simulink model "MS_QD2_QBPlat_R2021a"  (R2021a)
settings: Solver=ode2  StartTime=0.0  StopTime=inf  FixedStep=0.001  RelTol=1e-3  EnableMultiTasking=on
undefined symbols (not defined in the file): Host, localhost, qc_get_step_size
libraries: quarc_library x71, simulink x10, simulink_extras x2
(part 1 of 2)
settings Model: SimulationMode=external  ExtModeTrigDuration=10000  Creator=Admin  LastModifiedBy=jpineros
settings SolverCC: AlgebraicLoopSolver=TrustRegion  PositivePriorityOrder=on
settings DataIOCC: ReturnWorkspaceOutputs=off
settings DebuggingCC: SFUnexpectedBacktrackingDiag=warning  SFNoUnconditionalDefaultTransitionDiag=warning  SFExecutionAtInitializationDiag=none  ArithmeticOperatorsInVariantConditions=warning
settings SFSimCC: SimUseLocalCustomCode=off  CustomCodeUndefinedFunction=UseInterfaceOnly
settings RTWCC: Description=QUARC Win64 Target Using Toolchain  SystemTargetFile=quarc_win64.tlc  TemplateMakefile=quarc_default_tmf  RTWUseLocalCustomCode=off  Toolchain=QUARC win64 | nmake (64-bit Windows)  BuildConfiguration=Faster Runs
settings CodeAppCC: StateflowObjectComments=on
settings STFCustomTargetCC: ConcurrentExecutionCompliant=on  SystemTargetFile=quarc_win64.tlc
settings GRTTargetCC: TargetLangStandard=C89/C90 (ANSI)  ParMdlRefBuildCompliant=off  CompOptLevelCompliant=off  CombineOutputUpdateFcns=off  MatFileLogging=off  CPPClassGenCompliant=off  GRTInterface=on  ExtMode=on  ExtModeMexFile=quarc_comm  ExtModeMexArgs='-w -d %d -uri %u -drone_ip 192.168.2.11 -qbot_ip 192.168.2.21','tcpip://localhost:17001'
settings ConfigComp: CovMetricSettings=dw  CovSaveCumulativeToWorkspaceVar=on  CovSaveSingleToWorkspaceVar=on  CovExternalEMLEnable=off  CovBoundaryAbsTol=1.0e-5

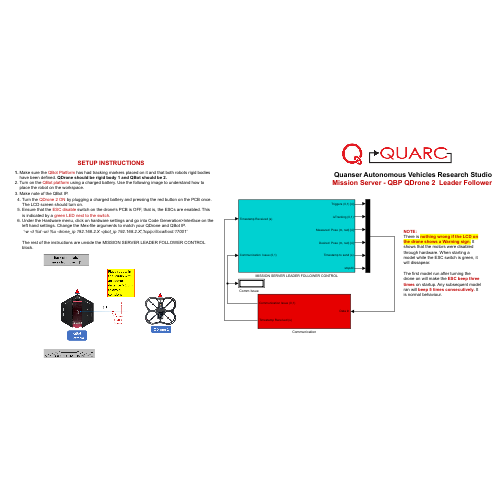
[thumbnail: Simulink's stored preview of the top-level diagram]
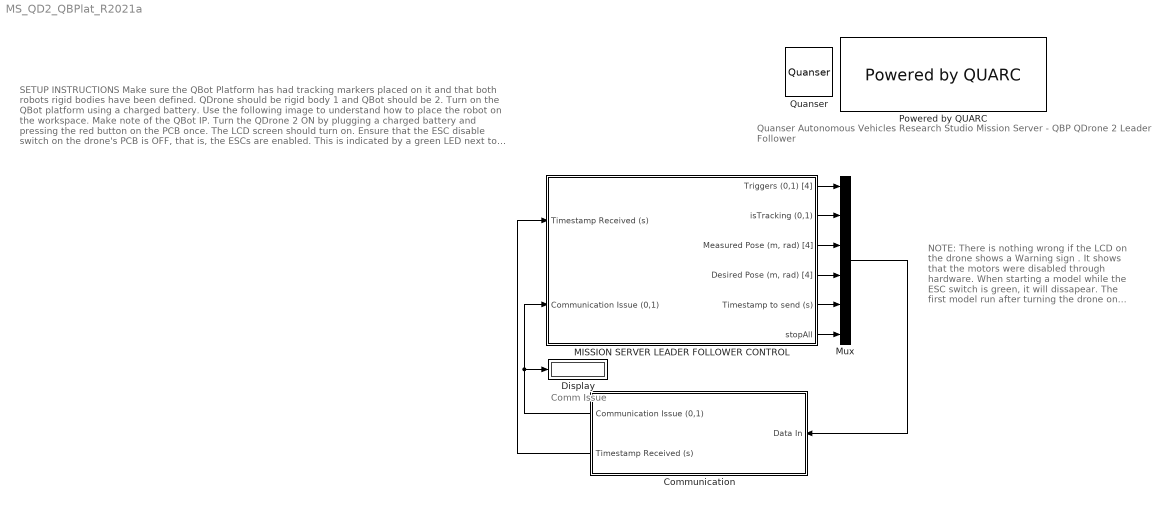
== system MS_QD2_QBPlat_R2021a ==
  note: Quanser Autonomous Vehicles Research Studio
      | Mission Server - QBP QDrone 2 Leader Follower
  note: Comm Issue
  note: NOTE:
      | There is nothing wrong if the LCD on the drone shows a Warning sign . It shows that the motors were disabled through hardware. When starting a model while the ESC switch is green, it will dissapear.
      |
      | The first model run after turning the drone on will make the ESC beep three times on startup. Any subsequent model ran will beep 5 times consecutively. It is normal behaviour.
  note: SETUP INSTRUCTIONS
      |
      | Make sure the QBot Platform has had tracking markers placed on it and that both robots rigid bodies have been defined. QDrone should be rigid body 1 and QBot should be 2.
      | Turn on the QBot platform using a charged battery. Use the following image to understand how to place the robot on the workspace.
      | Make note of the QBot IP.
      | Turn the QDrone 2 ON by plugging a charged battery and pressing the red button on the PCB once. The LCD screen should turn on.
      | Ensure that the ESC disable switch on the drone's PCB is OFF, that is, the ESCs are enabled. This is indicated by a green LED next to the switch .
      | Under the Hardware menu, click on hardware settings and go into Code Generation>Interface on the left hand settings. Change the Mex-file arguments to match your QDrone and QBot IP.
      | '-w -d %d -uri %u -drone_ip 192.168.2.X -qbot_ip 192.168.2.X','tcpip://localhost:17001'
      |
      | The rest of the instructions are unside the MISSION SERVER LEADER FOLLOWER CONTROL block.
  Communication : Subsystem
  Display : Display
  MISSION SERVER LEADER FOLLOWER CONTROL : Subsystem
  Mux : Mux  Inputs=6
  Powered by QUARC : quarc_library/Logos/Powered by QUARC
  Quanser : quarc_library/Logos/Quanser
  wires:
  Communication/2(Timestamp Received (s)) -> MISSION SERVER LEADER FOLLOWER CONTROL/1(Timestamp Received (s))
  MISSION SERVER LEADER FOLLOWER CONTROL/5(Timestamp to send (s)) -> Mux/5
  Mux/1 -> Communication/1(Data In)
  Communication/1(Communication Issue (0,1)) -> MISSION SERVER LEADER FOLLOWER CONTROL/2(Communication Issue (0,1)), Display/1
  MISSION SERVER LEADER FOLLOWER CONTROL/3("Measured Pose (m, rad) [4]") -> Mux/3
  MISSION SERVER LEADER FOLLOWER CONTROL/4("Desired Pose (m, rad) [4]") -> Mux/4
  MISSION SERVER LEADER FOLLOWER CONTROL/1(Triggers (0,1) [4]) -> Mux/1
  MISSION SERVER LEADER FOLLOWER CONTROL/2(isTracking (0,1)) -> Mux/2
  MISSION SERVER LEADER FOLLOWER CONTROL/6(stopAll) -> Mux/6

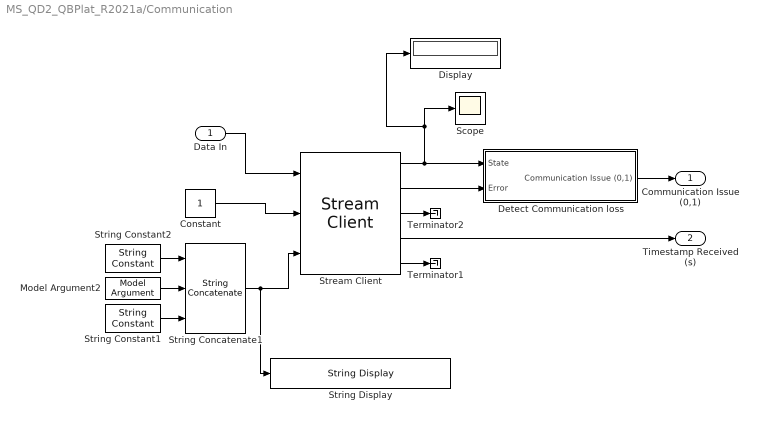
== system MS_QD2_QBPlat_R2021a/Communication ==
  Data In : Inport
  Constant : Constant
  Detect Communication loss : Subsystem
  Display : Display
  Model Argument2 : quarc_library/Sources/Signals/Model Argument  argument_name=drone_ip  has_value=on  data_type_mode=Specify via dialog  data_type=char  max_length=80  default_value=0  default_string=192.168.2.11  variable_size=off
      settings: AttributesFormatString=(-%<argument_name>)  SourceProductName=QUARC Targets
  Scope : Scope
  Stream Client : quarc_library/Communications/Basic/Stream Client  uri_source=External input port  uri=tcpip://192.168.2.11:18011  send_buffer_size=1460  receive_buffer_size=1460  byte_order=little endian (Intel - LSB first)  optimization=Minimum latency  send_options=Send most recent data  receive_options=Receive most recent data  default_value=zeros(1,1)  sample_time=qc_get_step_size  active=off  implementation=Use blocking I/O in a separate thread  send_fifo_size=1000  receive_fifo_size=1000  send_priority=0  receive_priority=0  send_dimensions=off  receive_dimensions=off  max_dimensions=-1  data_type=Inherited via back propagation  type_expr=BusObject
  String Concatenate1 : quarc_library/Strings/String Concatenate  num_inputs=3  max_length=0  output_size=Inherit from input
      settings: SourceProductName=QUARC Targets
  String Constant1 : quarc_library/Strings/String Constant  string_value=:18011?nagle='off'  evaluate_string=off  string_type=text  max_length=80  sample_time=inf  variable_size=off
      settings: AttributesFormatString="\":18011?nagle='off'\""  SourceProductName=QUARC Targets
  String Constant2 : quarc_library/Strings/String Constant  string_value=tcpip://  evaluate_string=off  string_type=text  max_length=80  sample_time=inf  variable_size=off
      settings: AttributesFormatString="\"tcpip://\""  SourceProductName=QUARC Targets
  String Display : quarc_library/Strings/String Display  alignment=center  display_mode=Single line  sample_time=-1  use_new=off
      settings: SourceProductName=QUARC Targets
  Terminator1 : Terminator
  Terminator2 : Terminator
  Communication Issue (0,1) : Outport  VectorParamsAs1DForOutWhenUnconnected=off
  Timestamp Received (s) : Outport  Port=2  VectorParamsAs1DForOutWhenUnconnected=off
  wires:
  Constant/1 -> Stream Client/2
  Data In/1 -> Stream Client/1
  Stream Client/3 -> Terminator2/1
  Stream Client/5 -> Terminator1/1
  Stream Client/4 -> Timestamp Received (s)/1
  Stream Client/1 -> Display/1, Scope/1, Detect Communication loss/1(State)
  Stream Client/2 -> Detect Communication loss/2(Error)
  Detect Communication loss/1(Communication Issue (0,1)) -> Communication Issue (0,1)/1
  Model Argument2/1 -> String Concatenate1/2
  String Constant2/1 -> String Concatenate1/1
  String Concatenate1/1 -> Stream Client/3, String Display/1
  String Constant1/1 -> String Concatenate1/3

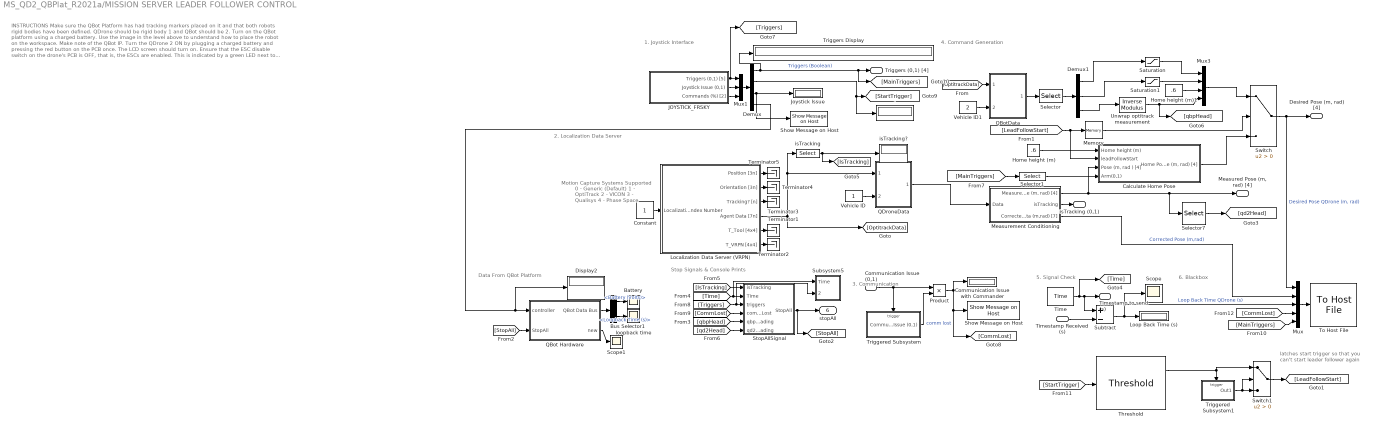
== system MS_QD2_QBPlat_R2021a/MISSION SERVER LEADER FOLLOWER CONTROL ==
  note: Data From QBot Platform
  note: Stop Signals & Console Prints
  note: latches start trigger so that you can't start leader follower again
  note: 5. Signal Check
  note: 6. Blackbox
  note: 3. Communication
  note: 2. Localization Data Server
  note: 1. Joystick Interface
  note: 4. Command Generation
  note: INSTRUCTIONS
      |
      | Make sure the QBot Platform has had tracking markers placed on it and that both robots rigid bodies have been defined. QDrone should be rigid body 1 and QBot should be 2.
      | Turn on the QBot platform using a charged battery. Use the image in the level above to understand how to place the robot on the workspace.
      | Make note of the QBot IP.
      | Turn the QDrone 2 ON by plugging a charged battery and pressing the red button on the PCB once. The LCD screen should turn on.
      | Ensure that the ESC disable switch on the drone's PCB is OFF, that is, the ESCs are enabled. This is indicated by a green LED next to the switch .
      | Under the Hrdware menu, click on hardware settings and go into Code Generation>Interface on the left hand settings. Change the Mex-file arguments to match your QDrone and QBot IP.
      | '-w -d %d -uri %u -drone_ip 192.168.2.X -qbot_ip 192.168.2.X','tcpip://localhost:17001'
      |
      | Open the Joystick subsystem and ensure that the Host Game Controller block's Controller Number parameter is set to FrSky Simulator THAT SUBSYSTEM ALSO WILL SHOW YOU HOW TO CONTROL THE SYSTEM USING THE DIFFERENT PARTS OF THE JOYSTICK
      | NOTE : In case of unexpected behaviour or emergencies, keep the Emergency Stop push button pressed on the joystick to cut all power to the motors (this will result in the drone falling).
      | Localization subsystem uses VRPN to communicate with third party motion capture systems. Change the motion capture system selector to the one currently used by your lab. Systems currently tested:
      | 0 - Generic (Default)
      | 1 - OptiTrack
      | 2 - VICON
      | 3 - Qualisys
      | 4 - Phase Space
      | Note: DO NOT change this number once the model has started.
      | Turn the Joystick ON and ensure all toggles are on the position away from you .
      | Under the HARDWARE menu, click on Monitor & Tune . Wait for the model to start running (takes ~1 to 5 seconds for the Motive API to initialize and send localization data).
      | In the MISSION CONTROL QDRONE POSITION CONTROL subsystem, ensure that the isTracking? display shows both values as 1 and that the Joystick Issue display shows 0 (joystick must be powered ON with USB dongle attached to the PC).
      | In your file explorer in the same folder as this file, right click on qbot_driver.rt-linux_qbot_platform and click on run on target.
      | Fill out the window that pops up as per the image underneath using the IP in the QBot's screen and click run. The LEDs of the QBot should changeto white.
      | Note: If you are used to running the qbot driver on startup for the QBot, stop the model and run this one instead. It has some modifications from the default QBot driver in other examples.
      | You should now be able to drive the QBot using the right joystick on the controller.
      |
      | In a new Matlab instance, open the QDrone.slx model and set the QDrone's IP in the Hardware Settings > Code Generation > Interface and click Monitor and drone. Wait for the Drone to beep.
      | Arm the drone by moving the Arm/Disarm toggle on the joystick to the 2 position. (Bringing it towards you). The props will start turning at a low speed.
      | Takeoff the drone by moving the Takeoff/Land toggle on the joystick to the 2 position (Bringing it towards you). The QDrone should takeoff and hover.
      | Switch the Leader Follower Start toggle (toggle on the right front of the joystick, use the image inside the joystick subsystem as a reference) towards you and the QDrone will start following above the QBot.
      | Drive the QBot with the joystick in the controller. The drone will fly only 1 meter on each direction of the origin, so if the qbot exits that area, the QDrone will stay behind but pointed towards the qbot.
      | Once done, switch the Leader follower Start toggle back to the starting position away from you and the QDrone will stay at its current position. Use the joystick to move the QBot away from under the QDrone.
      | When the QBot is safely away from the Drone, move the Takeoff/Land toggle on the joystick to the 0 position to land the drone. The QDrone should land.
      | Move the Arm/Disarm toggle on the joystick to the 0 position. (The QDrone.slx model disarms the drone and stops automatically upon landing).
      | Stop this model.
  note: Motion Capture Systems Supported
  note: 0 - Generic (Default)
      | 1 - OptiTrack
      | 2 - VICON
      | 3 - Qualisys
      | 4 - Phase Space
  Timestamp Received (s) : Inport
  Communication Issue (0,1) : Inport  Port=2
  . : Display
  Battery : Scope
  Bus Selector1 : BusSelector  OutputSignals=Battery (Volts),Loopback Time (s)
  Calculate Home Pose : Subsystem
  Communication Issue with Commander : Display
  Constant : Constant
  Demux : Demux  Outputs=[4 1 1 2]
  Demux1 : Demux  Outputs=3
  Display2 : Display
  Home height (m) : Constant  Value=.6
  Home height (m)1 : Constant  Value=.6
  JOYSTICK_FRSKY : Subsystem
      mask Display: image('frsky.jpg');
  Joystick Issue : Display
  "Localization Data Server (VRPN) " : Subsystem
  Loop Back Time (s) : Display
  Measurement Conditioning : Subsystem
  Memory : Memory
  Mux : Mux  Inputs=5
  Mux1 : Mux  Inputs=[5 1 2]
  Mux3 : Mux
  Product : Product
  QBot Hardware : Subsystem
  QBotData : Subsystem
  QDroneData : Subsystem
  Saturation : Saturate  UpperLimit=1  LowerLimit=-1
  Saturation1 : Saturate  UpperLimit=1  LowerLimit=-1
  Scope : Scope
  Scope1 : Scope
  Selector : Selector  InputPortWidth=7  IndexOptions=Index vector (dialog)  Indices=[1 2 6]  OutputSizes=1
  Selector1 : Selector  InputPortWidth=4  IndexOptions=Index vector (dialog)  Indices=[1]  OutputSizes=1
  Selector7 : Selector  InputPortWidth=4  IndexOptions=Index vector (dialog)  Indices=[4]  OutputSizes=1
  Show Message on Host : quarc_library/Sinks/Error Handling/Show Message on Host  message_type=Fixed error message  message_icon=Warning  message=Mission Server: Communication Issue with QDrone
      settings: AttributesFormatString="\"%<message>\""  SourceProductName=QUARC Targets
  "Show Message on Host " : quarc_library/Sinks/Error Handling/Show Message on Host  message_type=Fixed error message  message_icon=Warning  message=Mission Server: Joystick Disconnected
      settings: AttributesFormatString="\"%<message>\""  SourceProductName=QUARC Targets
  StopAllSignal : Subsystem
  Subsystem5 : Subsystem
  Subtract : Sum  Inputs=+-
  Switch : Switch  Criteria=u2 > Threshold
  Switch1 : Switch  Criteria=u2 > Threshold
  Terminator{1..5} (5 alike) : Terminator
  Threshold : quarc_library/Discontinuities/Threshold  operator=>  param_src=Specify via dialog  threshold=0  duration=0.1
      settings: SourceProductName=QUARC Targets
  Time : quarc_library/Sources/Time/Time  time_source=Wall clock  sample_time=qc_get_step_size
  To Host File : quarc_library/Sinks/To Host/To Host File  source=Specify via dialog (do not evaluate)  file_name=saved_data/%m/Mission_Server_%{date}_%{time}.mat  variable_name=mission_server_data  decimation=1  sample_time=-1  file_format=MAT-file v.5  options=No header or footer  append=off  final_file_name=saved_data/MS_QD2_QBPlat_R2021a_/Mission_Server_30-Sep-2026_09-51-03.mat  encoding=Default  bitrate=2000000
  Triggered Subsystem1 : Subsystem  TreatAsAtomicUnit=on
  Triggered Subsystem : Subsystem  TreatAsAtomicUnit=on
  Triggers Display : Display
  Unwrap optitrack measurement : quarc_library/Discontinuities/Inverse Modulus  modulus=2*pi  output_derivative=off  output_revolutions=off  max_x=Inf  min_x=-Inf
  Vehicle ID : Constant
  Vehicle ID1 : Constant  Value=2
  isTracking : Selector  InputPortWidth=14  IndexOptions=Index vector (dialog)  Indices=[7 14]  OutputSizes=1
  isTracking? : Display
  loopback time : Scope
  Triggers (0,1) [4] : Outport  VectorParamsAs1DForOutWhenUnconnected=off
  isTracking (0,1) : Outport  Port=2  VectorParamsAs1DForOutWhenUnconnected=off
  "Measured Pose (m, rad) [4]" : Outport  Port=3  VectorParamsAs1DForOutWhenUnconnected=off
  "Desired Pose (m, rad) [4]" : Outport  Port=4  VectorParamsAs1DForOutWhenUnconnected=off
  Timestamp to send (s) : Outport  Port=5  VectorParamsAs1DForOutWhenUnconnected=off
  stopAll : Outport  Port=6
  wires:
  Communication Issue (0,1)/1 -> Product/1, Triggered Subsystem/Trigger
  isTracking/1 -> isTracking?/1, [IsTracking]
  Demux/3 -> Joystick Issue/1, "Show Message on Host "/1
  Demux/1 -> Triggers (0,1) [4]/1, [MainTriggers], Triggers Display/1  "Triggers (Boolean)"
  Time/1 -> [Time], Subtract/1, Timestamp to send (s)/1
  Timestamp Received (s)/1 -> Subtract/2
  Subtract/1 -> Mux/3, Scope/1, Loop Back Time (s)/1  "Loop Back Time QDrone (s)"
  Switch/1 -> Mux/1, "Desired Pose (m, rad) [4]"/1  "Desired Pose QDrone (m, rad)"
  Measurement Conditioning/2(isTracking) -> isTracking (0,1)/1
  Vehicle ID/1 -> QDroneData/2(Vehicle ID)
  QDroneData/1(Vehicle Data) -> Measurement Conditioning/1(Data)
  Home height (m)/1 -> Calculate Home Pose/1(Home height (m))
  Triggered Subsystem/1(Communication Issue (0,1)) -> Product/2
  Product/1 -> Communication Issue with Commander/1, [CommLost], Show Message on Host/1  "comm lost"
  Mux/1 -> To Host File/1
  Selector1/1 -> Calculate Home Pose/4(Arm(0,1))
  Measurement Conditioning/1("Measured Pose (m, rad) [4]") -> Calculate Home Pose/3("Pose (m, rad ) [4]"), "Measured Pose (m, rad) [4]"/1, Selector7/1
  Measurement Conditioning/3(Corrected Pose Data (m,rad) [7]) -> Mux/2  "Corrected Pose (m,rad)"
  Mux1/1 -> Demux/1
  Calculate Home Pose/1("Home Pose (m, rad) [4]") -> Switch/3
  [LeadFollowStart] -> Calculate Home Pose/2(leadFollowStart), Memory/1
  JOYSTICK_FRSKY/2(Joystick Issue (0,1)) -> Mux1/2
  JOYSTICK_FRSKY/1(Triggers (0,1) [5]) -> [Triggers], Mux1/1
  JOYSTICK_FRSKY/3(Commands (%) [2]) -> Mux1/3
  Vehicle ID1/1 -> QBotData/2(Vehicle ID)
  QBotData/1(Vehicle Data) -> Selector/1
  Selector/1 -> Demux1/1
  Demux1/1 -> Saturation/1
  Demux1/2 -> Saturation1/1
  Demux1/3 -> Unwrap optitrack measurement/1
  Home height (m)1/1 -> Mux3/3
  Mux3/1 -> Switch/1
  Unwrap optitrack measurement/1 -> [qbpHead], Mux3/4
  Saturation/1 -> Mux3/1
  Saturation1/1 -> Mux3/2
  [OptitrackData] -> QBotData/1(Optitrack Data)
  QBot Hardware/1(QBot Data Bus) -> Bus Selector1/1
  Demux/2 -> ./1, [StartTrigger]
  Demux/4 -> QBot Hardware/1(controller), Display2/1
  QBot Hardware/2(new) -> Scope1/1
  [StopAll] -> QBot Hardware/2(StopAll)
  Memory/1 -> Switch/2
  StopAllSignal/1(StopAll) -> stopAll/1, [StopAll]
  [Triggers] -> StopAllSignal/3(triggers), Subsystem5/2(Triggers)
  [Time] -> StopAllSignal/2(Time), Subsystem5/1(Time)
  [IsTracking] -> StopAllSignal/1(isTracking)
  [CommLost] -> StopAllSignal/4(commLost)
  [qbpHead] -> StopAllSignal/5(qbpHeading)
  [qd2Head] -> StopAllSignal/6(qd2Heading)
  Selector7/1 -> [qd2Head]
  Switch1/1 -> [LeadFollowStart]
  Triggered Subsystem1/1(Out1) -> Switch1/2, Switch1/3
  Threshold/1 -> Switch1/1, Triggered Subsystem1/Trigger
  [CommLost] -> Mux/4
  [MainTriggers] -> Selector1/1
  [MainTriggers] -> Mux/5
  Bus Selector1/1 -> Battery/1  "<Battery (Volts)>"
  Bus Selector1/2 -> loopback time/1  "<Loopback Time (s)>"
  "Localization Data Server (VRPN) "/6(T_VRPN [4x4]) -> Terminator2/1
  Constant/1 -> "Localization Data Server (VRPN) "/1(Localization System Index Number)
  "Localization Data Server (VRPN) "/5(T_Tool [4x4]) -> Terminator1/1
  "Localization Data Server (VRPN) "/4(Agent Data [7n]) -> QDroneData/1(Optitrack Data), isTracking/1, [OptitrackData]
  "Localization Data Server (VRPN) "/3(Tracking? [n]) -> Terminator3/1
  "Localization Data Server (VRPN) "/2(Orientation [3n]) -> Terminator4/1
  "Localization Data Server (VRPN) "/1(Position [3n]) -> Terminator5/1
  [StartTrigger] -> Threshold/1

== system MS_QD2_QBPlat_R2021a/Communication/Detect Communication loss ==
  note: Check if stream is 2 (connected) and error is positive (error codes are negative). Otherwise issue a communication error.
  State : Inport
  Error : Inport  Port=2
  Data Type Conversion : DataTypeConversion
  MATLAB Function : MATLAB Function  TreatAsAtomicUnit=on
  Terminator2 : Terminator
  Threshold : quarc_library/Discontinuities/Threshold  operator=>=  param_src=Specify via dialog  threshold=0.5  duration=0.1
      settings: SourceProductName=QUARC Targets
  Time : quarc_library/Sources/Time/Time  time_source=Wall clock  sample_time=qc_get_step_size
  Communication Issue (0,1) : Outport  VectorParamsAs1DForOutWhenUnconnected=off
  wires:
  Error/1 -> MATLAB Function/3(error)
  MATLAB Function/1(stream_connection_loss) -> Threshold/1
  State/1 -> MATLAB Function/2(state)
  Time/1 -> MATLAB Function/1(time)
  Threshold/2 -> Terminator2/1
  Data Type Conversion/1 -> Communication Issue (0,1)/1
  Threshold/1 -> Data Type Conversion/1

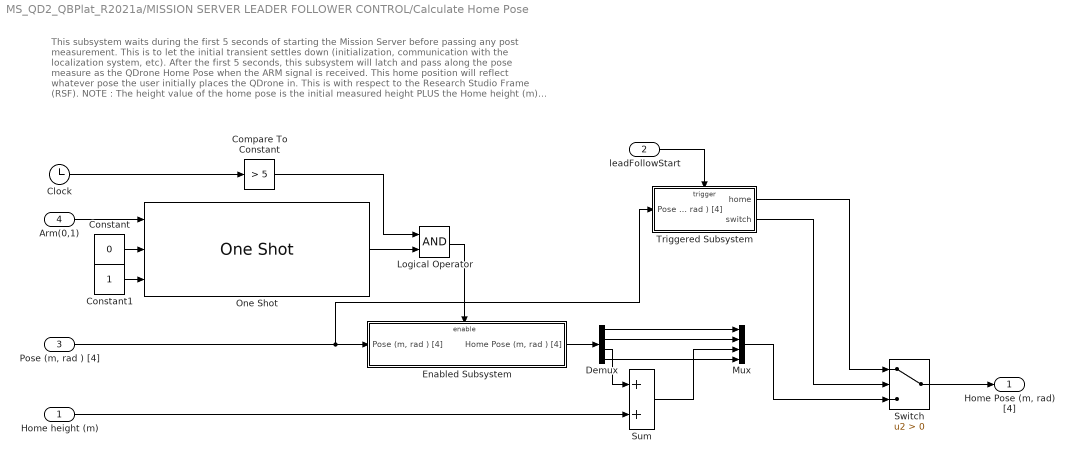
== system MS_QD2_QBPlat_R2021a/MISSION SERVER LEADER FOLLOWER CONTROL/Calculate Home Pose ==
  note: This subsystem waits during the first 5 seconds of starting the Mission Server before passing any post measurement.
      | This is to let the initial transient settles down (initialization, communication with the localization system, etc).
      | After the first 5 seconds, this subsystem will latch and pass along the pose measure as the QDrone Home Pose when
      | the ARM signal is received.
      | This home position will reflect whatever pose the user initially places the QDrone in.
      | This is with respect to the Research Studio Frame (RSF).
      |
      | NOTE : The height value of the home pose is the initial measured height PLUS the Home height (m) input value.
  Home height (m) : Inport
  leadFollowStart : Inport  Port=2
  "Pose (m, rad ) [4]" : Inport  Port=3
  Arm(0,1) : Inport  Port=4
  Clock : Clock
  Compare To Constant : simulink/Logic and Bit Operations/Compare To Constant  relop=>  const=5  OutDataTypeStr=boolean
  Constant : Constant  Value=0
  Constant1 : Constant
  Demux : Demux
  Enabled Subsystem : Subsystem  TreatAsAtomicUnit=on
  Logical Operator : Logic  AllPortsSameDT=off  OutDataTypeStr=boolean
  Mux : Mux
  One Shot : quarc_library/Discontinuities/One Shot  trigger_type=Rising edge  redun_pulse=Ignore extraneous pulse  width_source=Specify via dialog  pulse_width=1/qc_get_step_size
      settings: SourceProductName=QUARC Targets
  Sum : Sum
  Switch : Switch  Criteria=u2 > Threshold
  Triggered Subsystem : Subsystem  TreatAsAtomicUnit=on
  "Home Pose (m, rad) [4]" : Outport  VectorParamsAs1DForOutWhenUnconnected=off
  wires:
  Constant/1 -> One Shot/2
  Constant1/1 -> One Shot/3
  Arm(0,1)/1 -> One Shot/1
  One Shot/1 -> Logical Operator/2
  "Pose (m, rad ) [4]"/1 -> Enabled Subsystem/1("Pose (m, rad ) [4] "), Triggered Subsystem/1("Pose (m, rad ) [4]")
  Clock/1 -> Compare To Constant/1
  Compare To Constant/1 -> Logical Operator/1
  Enabled Subsystem/1("Home Pose (m, rad ) [4]") -> Demux/1
  Demux/1 -> Mux/1
  Demux/2 -> Mux/2
  Demux/3 -> Sum/1
  Sum/1 -> Mux/3
  Home height (m)/1 -> Sum/2
  Mux/1 -> Switch/3
  Logical Operator/1 -> Enabled Subsystem/Enable
  Demux/4 -> Mux/4
  Switch/1 -> "Home Pose (m, rad) [4]"/1
  Triggered Subsystem/2(switch) -> Switch/2
  leadFollowStart/1 -> Triggered Subsystem/Trigger
  Triggered Subsystem/1(home) -> Switch/1

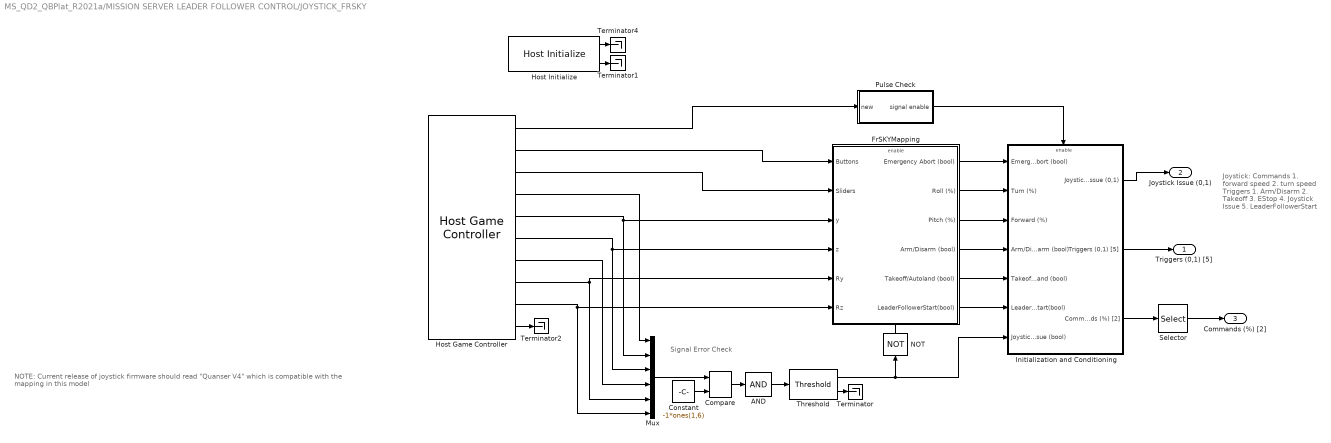
== system MS_QD2_QBPlat_R2021a/MISSION SERVER LEADER FOLLOWER CONTROL/JOYSTICK_FRSKY ==
  note: Signal Error Check
  note: NOTE: Current release of joystick firmware should read "Quanser V4" which is compatible with the mapping in this model
  note: Joystick:
      | Commands
      | 	1. forward speed
      | 	2. turn speed
      | Triggers
      | 	1. Arm/Disarm
      | 	2. Takeoff
      | 	3. EStop
      | 	4. Joystick Issue
      |
      | 	5. LeaderFollowerStart
  AND : Logic  Inputs=1  AllPortsSameDT=off  OutDataTypeStr=boolean
  Compare : quarc_library/Logic Operations/Compare  operator===  output_data_type=boolean
      settings: SourceProductName=QUARC Targets
  Constant : Constant  Value=-1*ones(1,6)
  FrSKYMapping : Subsystem
  Host Game Controller : quarc_library/Devices/Peripherals/Host/Host Game Controller  object_name=Host-1  controller=1  buffer_size=20  deadzone=[]  saturation=[]  sample_time=qc_get_step_size  auto_center=off  enabled=on  debug_mode=off
      settings: SourceProductName=QUARC Targets
  Host Initialize : quarc_library/Devices/Peripherals/Host/Host Initialize  object_name=Host-1  uri_source=Specify via dialog (do not evaluate)  uri=tcpip://localhost:18005  send_buffer_size=1000  receive_buffer_size=1000  thread_priority=0  run_client=on  use_window=off  window_position=[]  sample_time=qc_get_step_size  active=on
      settings: AttributesFormatString="\"tcpip://localhost:18005\""  SourceProductName=QUARC Targets
  Initialization and Conditioning : Subsystem  TreatAsAtomicUnit=on
  Mux : Mux  Inputs=6
  NOT : Logic  Operator=NOT  IconShape=distinctive  AllPortsSameDT=off  OutDataTypeStr=boolean
  Pulse Check : Subsystem  TreatAsAtomicUnit=on
  Selector : Selector  InputPortWidth=2  IndexOptions=Index vector (dialog)  Indices=[2 1]  OutputSizes=1
  Terminator{,1..2,4} (4 alike) : Terminator
  Threshold : quarc_library/Discontinuities/Threshold  operator=>=  param_src=Specify via dialog  threshold=0.5  duration=0.2
      settings: SourceProductName=QUARC Targets
  Triggers (0,1) [5] : Outport  VectorParamsAs1DForOutWhenUnconnected=off
  Joystick Issue (0,1) : Outport  Port=2  VectorParamsAs1DForOutWhenUnconnected=off
  Commands (%) [2] : Outport  Port=3  VectorParamsAs1DForOutWhenUnconnected=off
  wires:
  Host Game Controller/10 -> Terminator2/1
  Pulse Check/1(signal enable) -> Initialization and Conditioning/Enable
  Host Initialize/1 -> Terminator4/1
  FrSKYMapping/4("Arm/Disarm (bool) ") -> Initialization and Conditioning/4(Arm/Disarm (bool))
  Host Initialize/2 -> Terminator1/1
  FrSKYMapping/5(Takeoff/Autoland (bool)) -> Initialization and Conditioning/5(Takeoff/AutoLand (bool))
  Host Game Controller/7 -> Mux/4
  Host Game Controller/8 -> Mux/5, FrSKYMapping/5(Ry)
  Initialization and Conditioning/3(Commands (%) [2]) -> Selector/1
  Host Game Controller/5 -> Mux/2, FrSKYMapping/3(y)
  Host Game Controller/9 -> Mux/6, FrSKYMapping/6(Rz)
  Host Game Controller/1 -> Pulse Check/1(new)
  Mux/1 -> Compare/1
  Threshold/1 -> NOT/1, Initialization and Conditioning/7(Joystick Issue (bool))
  AND/1 -> Threshold/1
  Host Game Controller/3 -> FrSKYMapping/2(Sliders)
  Threshold/2 -> Terminator/1
  NOT/1 -> FrSKYMapping/Enable
  Constant/1 -> Compare/2
  Host Game Controller/6 -> Mux/3, FrSKYMapping/4(z)
  FrSKYMapping/2(Roll (%)) -> Initialization and Conditioning/2(Turn (%))
  FrSKYMapping/3(Pitch (%)) -> Initialization and Conditioning/3(Forward (%))
  Compare/1 -> AND/1
  FrSKYMapping/1(Emergency Abort (bool)) -> Initialization and Conditioning/1(Emergency Abort (bool))
  Initialization and Conditioning/1(Joystick Issue (0,1)) -> Joystick Issue (0,1)/1
  Initialization and Conditioning/2(Triggers (0,1) [5]) -> Triggers (0,1) [5]/1
  Host Game Controller/4 -> Mux/1
  Host Game Controller/2 -> FrSKYMapping/1(Buttons)
  FrSKYMapping/6(LeaderFollowerStart(bool)) -> Initialization and Conditioning/6(LeaderFollowerStart(bool))
  Selector/1 -> Commands (%) [2]/1

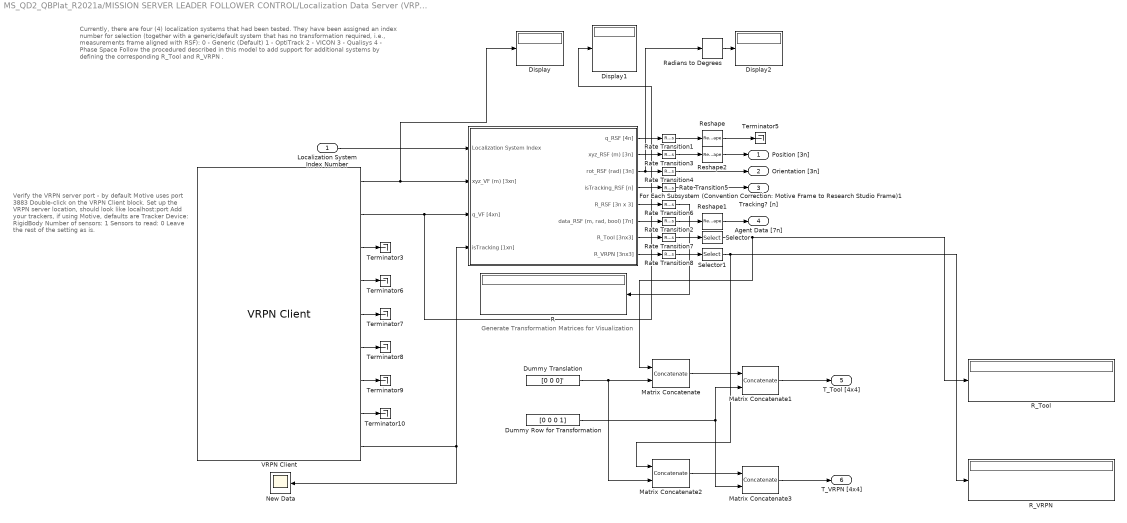
== system MS_QD2_QBPlat_R2021a/MISSION SERVER LEADER FOLLOWER CONTROL/Localization Data Server (VRPN)  ==
  note: Generate Transformation Matrices for Visualization
  note: Verify the VRPN server port - by default Motive uses port 3883
      | Double-click on the VRPN Client block.
      |
      | Set up the VRPN server location, should look like
      | localhost:port
      |
      | Add your trackers,
      | if using Motive, defaults are
      | Tracker Device: RigidBody
      | Number of sensors: 1
      | Sensors to read: 0
      |
      | Leave the rest of the setting as is.
  note: Currently, there are four (4) localization systems that had been tested. They have been assigned an index number for selection (together with a generic/default system that has no transformation required, i.e., measurements frame aligned with RSF):
      |
      | 0 - Generic (Default)
      | 1 - OptiTrack
      | 2 - VICON
      | 3 - Qualisys
      | 4 - Phase Space
      |
      | Follow the procedured described in this model to add support for additional systems by defining the corresponding R_Tool and R_VRPN .
  Localization System Index Number : Inport
  Display : Display
  Display1 : Display
  Display2 : Display
  Dummy Row for Transformation : Constant  Value=[0 0 0 1]  VectorParams1D=off
  Dummy Translation : Constant  Value=[0 0 0]'  VectorParams1D=off
  For Each Subsystem (Convention Correction: Motive Frame to Research Studio Frame)1 : Subsystem  TreatAsAtomicUnit=on
  Matrix Concatenate : Concatenate  Mode=Multidimensional array  ConcatenateDimension=2
  Matrix Concatenate1 : Concatenate  Mode=Multidimensional array
  Matrix Concatenate2 : Concatenate  Mode=Multidimensional array  ConcatenateDimension=2
  Matrix Concatenate3 : Concatenate  Mode=Multidimensional array
  New Data : Scope
  R : Display
  R_Tool : Display
  R_VRPN : Display
  Radians to Degrees : simulink_extras/Transformations/Radians to Degrees
  Rate Transition{1..8} (8 alike) : RateTransition
  Reshape : Reshape
  Reshape1 : Reshape
  Reshape2 : Reshape
  Selector : Selector  NumberOfDimensions=2  InputPortWidth=3  IndexOptions=Index vector (dialog),Index vector (dialog)  Indices=[1:3],[1:3]  OutputSizes=1,1
  Selector1 : Selector  NumberOfDimensions=2  InputPortWidth=3  IndexOptions=Index vector (dialog),Index vector (dialog)  Indices=[1:3],[1:3]  OutputSizes=1,1
  Terminator{3,5..10} (7 alike) : Terminator
  VRPN Client : quarc_library/Devices/Third-Party/VRPN/VRPN Client  server_address=localhost:3883  trackerstable={ 'RigidBody1', '1', '0'; 'RigidBody2', '1', '0' }  trackers_list_mask='RigidBody1|RigidBody2'  trackers_num_sensors="[1  1]"  trackers_sensors_to_read_arg="[1  1  0  0]"  trackers_jpl=off  sample_time=qc_get_step_size*16  active=on
      settings: SourceProductName=QUARC Targets
  Position [3n] : Outport  VectorParamsAs1DForOutWhenUnconnected=off
  Orientation [3n] : Outport  Port=2  VectorParamsAs1DForOutWhenUnconnected=off
  Tracking? [n] : Outport  Port=3  VectorParamsAs1DForOutWhenUnconnected=off
  Agent Data [7n] : Outport  Port=4  VectorParamsAs1DForOutWhenUnconnected=off
  T_Tool [4x4] : Outport  Port=5  VectorParamsAs1DForOutWhenUnconnected=off
  T_VRPN [4x4] : Outport  Port=6  VectorParamsAs1DForOutWhenUnconnected=off
  wires:
  VRPN Client/1 -> Display/1, For Each Subsystem (Convention Correction: Motive Frame to Research Studio Frame)1/2(xyz_VF (m) [3xn])
  VRPN Client/2 -> Display1/1, For Each Subsystem (Convention Correction: Motive Frame to Research Studio Frame)1/3(q_VF [4xn])
  For Each Subsystem (Convention Correction: Motive Frame to Research Studio Frame)1/4(isTracking_RSF [n]) -> Rate Transition5/1
  For Each Subsystem (Convention Correction: Motive Frame to Research Studio Frame)1/3(rot_RSF (rad) [3n]) -> Radians to Degrees/1, Rate Transition4/1
  For Each Subsystem (Convention Correction: Motive Frame to Research Studio Frame)1/2(xyz_RSF (m) [3n]) -> Rate Transition3/1
  VRPN Client/3 -> Terminator3/1
  Reshape/1 -> Terminator5/1
  VRPN Client/4 -> Terminator6/1
  VRPN Client/5 -> Terminator7/1
  VRPN Client/6 -> Terminator8/1
  VRPN Client/7 -> Terminator9/1
  VRPN Client/8 -> Terminator10/1
  VRPN Client/9 -> For Each Subsystem (Convention Correction: Motive Frame to Research Studio Frame)1/4(isTracking [1xn]), New Data/1
  For Each Subsystem (Convention Correction: Motive Frame to Research Studio Frame)1/6("data_RSF (m, rad, bool) [7n]") -> Rate Transition2/1
  For Each Subsystem (Convention Correction: Motive Frame to Research Studio Frame)1/1(q_RSF [4n]) -> Rate Transition1/1
  Rate Transition2/1 -> Reshape1/1
  Rate Transition1/1 -> Reshape/1
  Reshape1/1 -> Agent Data [7n]/1
  Reshape2/1 -> Position [3n]/1
  Rate Transition3/1 -> Reshape2/1
  Rate Transition4/1 -> Orientation [3n]/1
  Rate Transition5/1 -> Tracking? [n]/1
  For Each Subsystem (Convention Correction: Motive Frame to Research Studio Frame)1/5(R_RSF [3n x 3]) -> Rate Transition6/1
  Rate Transition6/1 -> R/1
  Localization System Index Number/1 -> For Each Subsystem (Convention Correction: Motive Frame to Research Studio Frame)1/1(Localization System Index)
  For Each Subsystem (Convention Correction: Motive Frame to Research Studio Frame)1/7(R_Tool [3nx3]) -> Rate Transition7/1
  Rate Transition7/1 -> Selector/1
  Rate Transition8/1 -> Selector1/1
  For Each Subsystem (Convention Correction: Motive Frame to Research Studio Frame)1/8(R_VRPN [3nx3]) -> Rate Transition8/1
  Selector/1 -> Matrix Concatenate/1, R_Tool/1
  Dummy Translation/1 -> Matrix Concatenate2/2, Matrix Concatenate/2
  Matrix Concatenate/1 -> Matrix Concatenate1/1
  Matrix Concatenate1/1 -> T_Tool [4x4]/1
  Dummy Row for Transformation/1 -> Matrix Concatenate3/2, Matrix Concatenate1/2
  Matrix Concatenate2/1 -> Matrix Concatenate3/1
  Selector1/1 -> Matrix Concatenate2/1, R_VRPN/1
  Matrix Concatenate3/1 -> T_VRPN [4x4]/1
  Radians to Degrees/1 -> Display2/1

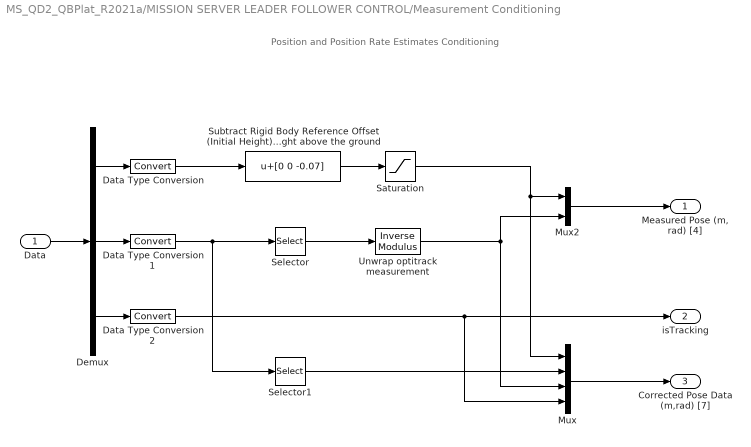
== system MS_QD2_QBPlat_R2021a/MISSION SERVER LEADER FOLLOWER CONTROL/Measurement Conditioning ==
  note: Position and Position Rate Estimates Conditioning
  Data : Inport
  Data Type Conversion : DataTypeConversion
  Data Type Conversion1 : DataTypeConversion
  Data Type Conversion2 : DataTypeConversion
  Demux : Demux  Outputs=[3 3 1]
  Mux : Mux
  Mux2 : Mux  Inputs=[3 1]
  Saturation : Saturate  UpperLimit=[2 2 5]  LowerLimit=[-2 -2 0]
  Selector : Selector  InputPortWidth=3  IndexOptions=Index vector (dialog)  Indices=[3]  OutputSizes=1
  Selector1 : Selector  InputPortWidth=3  IndexOptions=Index vector (dialog)  Indices=[1 2]  OutputSizes=1
  Subtract Rigid Body Reference Offset (Initial Height) to get height above the ground : Bias  Bias=[0 0 -0.07]
  Unwrap optitrack measurement : quarc_library/Discontinuities/Inverse Modulus  modulus=2*pi  output_derivative=off  output_revolutions=off  max_x=Inf  min_x=-Inf
  "Measured Pose (m, rad) [4]" : Outport  VectorParamsAs1DForOutWhenUnconnected=off
  isTracking : Outport  Port=2  VectorParamsAs1DForOutWhenUnconnected=off
  Corrected Pose Data (m,rad) [7] : Outport  Port=3  VectorParamsAs1DForOutWhenUnconnected=off
  wires:
  Demux/2 -> Data Type Conversion1/1
  Demux/1 -> Data Type Conversion/1
  Demux/3 -> Data Type Conversion2/1
  Mux2/1 -> "Measured Pose (m, rad) [4]"/1
  Data/1 -> Demux/1
  Data Type Conversion2/1 -> Mux/4, isTracking/1
  Subtract Rigid Body Reference Offset (Initial Height) to get height above the ground/1 -> Saturation/1
  Saturation/1 -> Mux2/1, Mux/1
  Data Type Conversion1/1 -> Selector1/1, Selector/1
  Selector/1 -> Unwrap optitrack measurement/1
  Data Type Conversion/1 -> Subtract Rigid Body Reference Offset (Initial Height) to get height above the ground/1
  Unwrap optitrack measurement/1 -> Mux/3, Mux2/2
  Mux/1 -> Corrected Pose Data (m,rad) [7]/1
  Selector1/1 -> Mux/2

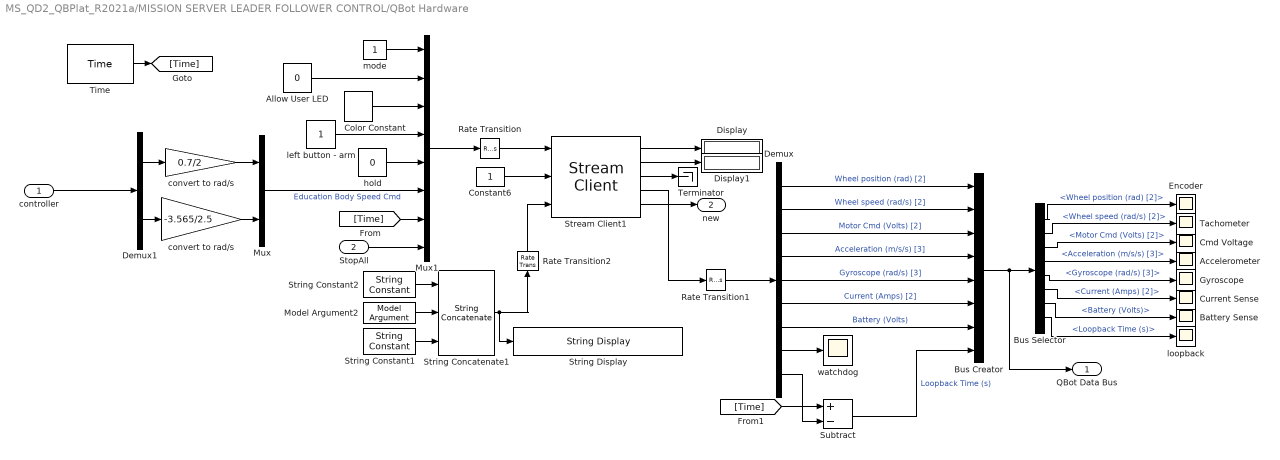
== system MS_QD2_QBPlat_R2021a/MISSION SERVER LEADER FOLLOWER CONTROL/QBot Hardware ==
  controller : Inport
  StopAll : Inport  Port=2
  Accelerometer : Scope
  Allow User LED : Constant  Value=0
  Battery Sense : Scope
  Bus Creator : BusCreator  Inputs=8
  Bus Selector : BusSelector  OutputSignals=Wheel position (rad) [2],Wheel speed (rad/s) [2],Motor Cmd (Volts) [2],Acceleration (m/s/s) [3],Gyroscope (rad/s) [3],Current (Amps) [2],Battery (Volts),Loopback Time (s)
  Cmd Voltage : Scope
  Color Constant : quarc_library/Sources/Signals/Color Constant  color=[0 1 1]
      settings: SourceProductName=QUARC Targets
  Constant6 : Constant
  Current Sense : Scope
  Demux : Demux  Outputs=[2 2 2 3 3 2 1 1 1]
  Demux1 : Demux  Outputs=2
  Display : Display
  Display1 : Display
  Encoder : Scope
  Gyroscope : Scope
  Model Argument2 : quarc_library/Sources/Signals/Model Argument  argument_name=qbot_ip  has_value=on  data_type_mode=Specify via dialog  data_type=char  max_length=80  default_value=0  default_string=192.168.2.21  variable_size=off
      settings: AttributesFormatString=(-%<argument_name>)  SourceProductName=QUARC Targets
  Mux : Mux  Inputs=2
  Mux1 : Mux  Inputs=8
  Rate Transition : RateTransition
  Rate Transition1 : RateTransition
  Rate Transition2 : RateTransition
  Stream Client1 : quarc_library/Communications/Basic/Stream Client  uri_source=External input port  uri=tcpip://192.168.2.21:18021  send_buffer_size=1460  receive_buffer_size=1460  byte_order=little endian (Intel - LSB first)  optimization=Minimum latency  send_options=Send most recent data  receive_options=Receive most recent data  default_value=zeros(17,1)  sample_time=qc_get_step_size * ceil(1/60 / qc_get_step_size)  active=off  implementation=Use blocking I/O in a separate thread  send_fifo_size=1000  receive_fifo_size=1000  send_priority=0  receive_priority=0  send_dimensions=off  receive_dimensions=off  max_dimensions=-1  data_type=Inherited via back propagation  type_expr=BusObject
  String Concatenate1 : quarc_library/Strings/String Concatenate  num_inputs=3  max_length=0  output_size=Inherit from input
      settings: SourceProductName=QUARC Targets
  String Constant1 : quarc_library/Strings/String Constant  string_value=:18021?nagle='off'  evaluate_string=off  string_type=text  max_length=80  sample_time=inf  variable_size=off
      settings: AttributesFormatString="\":18021?nagle='off'\""  SourceProductName=QUARC Targets
  String Constant2 : quarc_library/Strings/String Constant  string_value=tcpip://  evaluate_string=off  string_type=text  max_length=80  sample_time=inf  variable_size=off
      settings: AttributesFormatString="\"tcpip://\""  SourceProductName=QUARC Targets
  String Display : quarc_library/Strings/String Display  alignment=center  display_mode=Single line  sample_time=-1  use_new=off
      settings: SourceProductName=QUARC Targets
  Subtract : Sum  Inputs=+-
  Tachometer : Scope
  Terminator : Terminator
  Time : quarc_library/Sources/Time/Time  time_source=Wall clock  sample_time=qc_get_step_size
  convert to rad/s : Gain  Gain=0.7/2
  "convert to rad/s " : Gain  Gain=-3.565/2.5
  hold : Constant  Value=0
  left button - arm : Constant
  loopback : Scope
  mode : Constant
  watchdog : Scope
  QBot Data Bus : Outport
  new : Outport  Port=2
  wires:
  Demux/2 -> Bus Creator/2  "Wheel speed (rad/s) [2]"
  mode/1 -> Mux1/1
  Stream Client1/3 -> Terminator/1
  Stream Client1/1 -> Display/1
  Stream Client1/2 -> Display1/1
  Color Constant/1 -> Mux1/3
  Allow User LED/1 -> Mux1/2
  Demux/3 -> Bus Creator/3  "Motor Cmd (Volts) [2]"
  Mux1/1 -> Rate Transition/1
  Stream Client1/4 -> Rate Transition1/1
  Demux/1 -> Bus Creator/1  "Wheel position (rad) [2]"
  Stream Client1/5 -> new/1
  Demux/7 -> Bus Creator/7  "Battery (Volts)"
  Demux/5 -> Bus Creator/5  "Gyroscope (rad/s) [3]"
  Demux/6 -> Bus Creator/6  "Current (Amps) [2]"
  Demux/9 -> Subtract/2
  hold/1 -> Mux1/5
  Demux/4 -> Bus Creator/4  "Acceleration (m/s/s) [3]"
  left button - arm/1 -> Mux1/4
  Bus Creator/1 -> QBot Data Bus/1, Bus Selector/1
  Subtract/1 -> Bus Creator/8  "Loopback Time (s)"
  Demux/8 -> watchdog/1
  Demux1/2 -> "convert to rad/s "/1
  controller/1 -> Demux1/1
  convert to rad/s/1 -> Mux/1
  "convert to rad/s "/1 -> Mux/2
  Demux1/1 -> convert to rad/s/1
  Mux/1 -> Mux1/6  "Education Body Speed Cmd"
  Rate Transition/1 -> Stream Client1/1
  Rate Transition1/1 -> Demux/1
  Constant6/1 -> Stream Client1/2
  StopAll/1 -> Mux1/8
  String Constant2/1 -> String Concatenate1/1
  String Constant1/1 -> String Concatenate1/3
  Model Argument2/1 -> String Concatenate1/2
  String Concatenate1/1 -> Rate Transition2/1, String Display/1
  Time/1 -> [Time]
  [Time] -> Mux1/7
  [Time] -> Subtract/1
  Rate Transition2/1 -> Stream Client1/3
  Bus Selector/7 -> Battery Sense/1  "<Battery (Volts)>"
  Bus Selector/5 -> Gyroscope/1  "<Gyroscope (rad/s) [3]>"
  Bus Selector/6 -> Current Sense/1  "<Current (Amps) [2]>"
  Bus Selector/3 -> Cmd Voltage/1  "<Motor Cmd (Volts) [2]>"
  Bus Selector/4 -> Accelerometer/1  "<Acceleration (m/s/s) [3]>"
  Bus Selector/1 -> Encoder/1  "<Wheel position (rad) [2]>"
  Bus Selector/2 -> Tachometer/1  "<Wheel speed (rad/s) [2]>"
  Bus Selector/8 -> loopback/1  "<Loopback Time (s)>"

== system MS_QD2_QBPlat_R2021a/MISSION SERVER LEADER FOLLOWER CONTROL/QBotData ==
  Optitrack Data : Inport
  Vehicle ID : Inport  Port=2
  Data Type Conversion10 : DataTypeConversion
  Data Type Conversion11 : DataTypeConversion
  Data Type Conversion9 : DataTypeConversion
  Extract Object Data : MATLAB Function  TreatAsAtomicUnit=on
  Mux1 : Mux  Inputs=3
  Reshape : Reshape
  Reshape1 : Reshape
  Reshape2 : Reshape
  Vehicle Data : Outport  VectorParamsAs1DForOutWhenUnconnected=off
  wires:
  Reshape2/1 -> Data Type Conversion9/1
  Reshape1/1 -> Data Type Conversion10/1
  Reshape/1 -> Data Type Conversion11/1
  Data Type Conversion9/1 -> Mux1/3
  Data Type Conversion10/1 -> Mux1/2
  Data Type Conversion11/1 -> Mux1/1
  Extract Object Data/2(orientation) -> Reshape1/1
  Extract Object Data/3(tracking) -> Reshape2/1
  Extract Object Data/1(position) -> Reshape/1
  Mux1/1 -> Vehicle Data/1
  Optitrack Data/1 -> Extract Object Data/1(data)
  Vehicle ID/1 -> Extract Object Data/2(index)

== system MS_QD2_QBPlat_R2021a/MISSION SERVER LEADER FOLLOWER CONTROL/QDroneData ==
  Optitrack Data : Inport
  Vehicle ID : Inport  Port=2
  Data Type Conversion10 : DataTypeConversion
  Data Type Conversion11 : DataTypeConversion
  Data Type Conversion9 : DataTypeConversion
  Extract Object Data : MATLAB Function  TreatAsAtomicUnit=on
  Mux1 : Mux  Inputs=3
  Reshape : Reshape
  Reshape1 : Reshape
  Reshape2 : Reshape
  Vehicle Data : Outport  VectorParamsAs1DForOutWhenUnconnected=off
  wires:
  Vehicle ID/1 -> Extract Object Data/2(index)
  Optitrack Data/1 -> Extract Object Data/1(data)
  Mux1/1 -> Vehicle Data/1
  Extract Object Data/1(position) -> Reshape/1
  Extract Object Data/3(tracking) -> Reshape2/1
  Extract Object Data/2(orientation) -> Reshape1/1
  Data Type Conversion11/1 -> Mux1/1
  Data Type Conversion10/1 -> Mux1/2
  Data Type Conversion9/1 -> Mux1/3
  Reshape/1 -> Data Type Conversion11/1
  Reshape1/1 -> Data Type Conversion10/1
  Reshape2/1 -> Data Type Conversion9/1

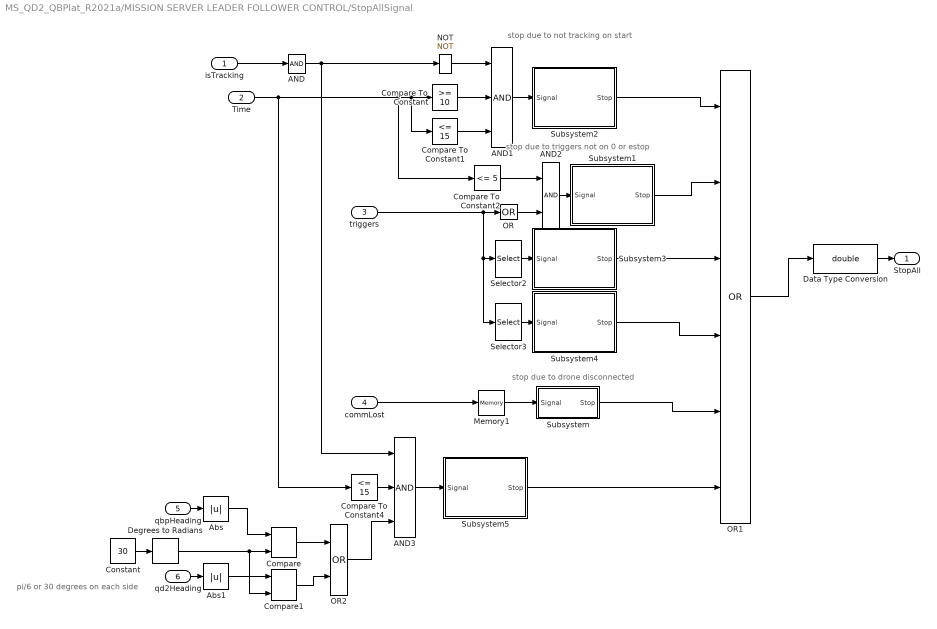
== system MS_QD2_QBPlat_R2021a/MISSION SERVER LEADER FOLLOWER CONTROL/StopAllSignal ==
  note: pi/6 or 30 degrees on each side
  note: stop due to not tracking on start
  note: stop due to triggers not on 0 or estop
  note: stop due to drone disconnected
  isTracking : Inport
  Time : Inport  Port=2
  triggers : Inport  Port=3
  commLost : Inport  Port=4
  qbpHeading : Inport  Port=5
  qd2Heading : Inport  Port=6
  AND : Logic  Inputs=1  IconShape=distinctive  AllPortsSameDT=off  OutDataTypeStr=boolean
  AND1 : Logic  Inputs=3  AllPortsSameDT=off  OutDataTypeStr=boolean
  AND2 : Logic  AllPortsSameDT=off  OutDataTypeStr=boolean
  AND3 : Logic  Inputs=3  AllPortsSameDT=off  OutDataTypeStr=boolean
  Abs : Abs
  Abs1 : Abs
  Compare : quarc_library/Logic Operations/Compare  operator=>=  output_data_type=boolean
      settings: SourceProductName=QUARC Targets
  Compare To Constant : simulink/Logic and Bit Operations/Compare To Constant  relop=>=  const=10  OutDataTypeStr=boolean
  Compare To Constant1 : simulink/Logic and Bit Operations/Compare To Constant  relop=<=  const=15  OutDataTypeStr=boolean
  Compare To Constant2 : simulink/Logic and Bit Operations/Compare To Constant  relop=<=  const=5  OutDataTypeStr=boolean
  Compare To Constant4 : simulink/Logic and Bit Operations/Compare To Constant  relop=<=  const=15  OutDataTypeStr=boolean
  Compare1 : quarc_library/Logic Operations/Compare  operator=>=  output_data_type=boolean
      settings: SourceProductName=QUARC Targets
  Constant : Constant  Value=30
  Data Type Conversion : DataTypeConversion  OutDataTypeStr=double
  Degrees to Radians : simulink_extras/Transformations/Degrees to Radians
  Memory1 : Memory
  NOT : Logic  Operator=NOT  IconShape=distinctive  AllPortsSameDT=off  OutDataTypeStr=boolean
  OR : Logic  Operator=OR  Inputs=1  IconShape=distinctive  AllPortsSameDT=off  OutDataTypeStr=boolean
  OR1 : Logic  Operator=OR  Inputs=6  AllPortsSameDT=off  OutDataTypeStr=boolean
  OR2 : Logic  Operator=OR  AllPortsSameDT=off  OutDataTypeStr=boolean
  Selector2 : Selector  InputPortWidth=5  IndexOptions=Index vector (dialog)  Indices=[3]  OutputSizes=1
  Selector3 : Selector  InputPortWidth=5  IndexOptions=Index vector (dialog)  Indices=[2]  OutputSizes=1
  Subsystem : Subsystem
  Subsystem1 : Subsystem
  Subsystem2 : Subsystem
  Subsystem3 : Subsystem
  Subsystem4 : Subsystem
  Subsystem5 : Subsystem
  StopAll : Outport
  wires:
  Compare To Constant1/1 -> AND1/3
  Subsystem/1(Stop) -> OR1/5
  Subsystem1/1(Stop) -> OR1/2
  Subsystem4/1(Stop) -> OR1/4
  OR1/1 -> Data Type Conversion/1
  triggers/1 -> OR/1, Selector3/1, Selector2/1
  AND1/1 -> Subsystem2/1(Signal)
  Selector2/1 -> Subsystem3/1(Signal)
  Subsystem2/1(Stop) -> OR1/1
  Selector3/1 -> Subsystem4/1(Signal)
  Memory1/1 -> Subsystem/1(Signal)
  commLost/1 -> Memory1/1
  AND2/1 -> Subsystem1/1(Signal)
  NOT/1 -> AND1/1
  Compare To Constant/1 -> AND1/2
  OR/1 -> AND2/2
  Subsystem3/1(Stop) -> OR1/3
  Compare To Constant2/1 -> AND2/1
  AND/1 -> NOT/1, AND3/1
  isTracking/1 -> AND/1
  Data Type Conversion/1 -> StopAll/1
  Time/1 -> Compare To Constant4/1, Compare To Constant2/1, Compare To Constant1/1, Compare To Constant/1
  Compare To Constant4/1 -> AND3/2
  qbpHeading/1 -> Abs/1
  qd2Heading/1 -> Abs1/1
  Abs/1 -> Compare/1
  Abs1/1 -> Compare1/1
  Compare/1 -> OR2/1
  Compare1/1 -> OR2/2
  OR2/1 -> AND3/3
  AND3/1 -> Subsystem5/1(Signal)
  Subsystem5/1(Stop) -> OR1/6
  Constant/1 -> Degrees to Radians/1
  Degrees to Radians/1 -> Compare1/2, Compare/2

== system MS_QD2_QBPlat_R2021a/MISSION SERVER LEADER FOLLOWER CONTROL/Subsystem5 ==
  Time : Inport
  Triggers : Inport  Port=2
  Demux2 : Demux  Outputs=5
  Triggered Subsystem1 : Subsystem  TreatAsAtomicUnit=on
  Triggered Subsystem2 : Subsystem  TreatAsAtomicUnit=on
  Triggered Subsystem3 : Subsystem  TreatAsAtomicUnit=on
  Triggered Subsystem4 : Subsystem  TreatAsAtomicUnit=on
  Triggered Subsystem5 : Subsystem  TreatAsAtomicUnit=on
  Triggered Subsystem6 : Subsystem  TreatAsAtomicUnit=on
  Triggered Subsystem7 : Subsystem  TreatAsAtomicUnit=on
  wires:
  Demux2/3 -> Triggered Subsystem3/Trigger
  Triggers/1 -> Demux2/1
  Demux2/5 -> Triggered Subsystem6/Trigger, Triggered Subsystem5/Trigger
  Demux2/2 -> Triggered Subsystem7/Trigger, Triggered Subsystem2/Trigger
  Demux2/1 -> Triggered Subsystem1/Trigger
  Demux2/4 -> Triggered Subsystem4/Trigger
  Time/1 -> Triggered Subsystem6/1(Time (s)), Triggered Subsystem5/1(Time (s)), Triggered Subsystem4/1(Time (s)), Triggered Subsystem3/1(Time (s)), Triggered Subsystem7/1(Time (s)), Triggered Subsystem2/1(Time (s)), Triggered Subsystem1/1(Time (s))

== system MS_QD2_QBPlat_R2021a/MISSION SERVER LEADER FOLLOWER CONTROL/Triggered Subsystem1 ==
  Trigger : TriggerPort  TriggerType=falling  VariantControl=(inherit)
  Constant : Constant  Value=0
  Out1 : Outport  InitialOutput=[1]
  wires:
  Constant/1 -> Out1/1

== system MS_QD2_QBPlat_R2021a/MISSION SERVER LEADER FOLLOWER CONTROL/Triggered Subsystem ==
  note: This looks for the first falling edge of the communication issue before allowing a communication issue to be triggered,
      | because the mission server model starts first.
  Trigger : TriggerPort  TriggerType=falling  VariantControl=Variant
  Add : Sum
  Compare To Constant : simulink/Logic and Bit Operations/Compare To Constant  relop=>=  const=1  OutDataTypeStr=boolean
  Constant : Constant
  Memory : Memory  InheritSampleTime=on
  Communication Issue (0,1) : Outport  InitialOutput=0  VectorParamsAs1DForOutWhenUnconnected=off
  wires:
  Constant/1 -> Add/1
  Memory/1 -> Add/2
  Add/1 -> Compare To Constant/1, Memory/1
  Compare To Constant/1 -> Communication Issue (0,1)/1

== system MS_QD2_QBPlat_R2021a/MISSION SERVER LEADER FOLLOWER CONTROL/Calculate Home Pose/Enabled Subsystem ==
  "Pose (m, rad ) [4] " : Inport
  Enable : EnablePort
  "Home Pose (m, rad ) [4]" : Outport  VectorParamsAs1DForOutWhenUnconnected=off
  wires:
  "Pose (m, rad ) [4] "/1 -> "Home Pose (m, rad ) [4]"/1

== system MS_QD2_QBPlat_R2021a/MISSION SERVER LEADER FOLLOWER CONTROL/Calculate Home Pose/Triggered Subsystem ==
  "Pose (m, rad ) [4]" : Inport
  Trigger : TriggerPort  TriggerType=falling  VariantControl=(inherit)
  Constant : Constant
  home : Outport  InitialOutput=[0]
  switch : Outport  Port=2  InitialOutput=[0]
  wires:
  Constant/1 -> switch/1
  "Pose (m, rad ) [4]"/1 -> home/1

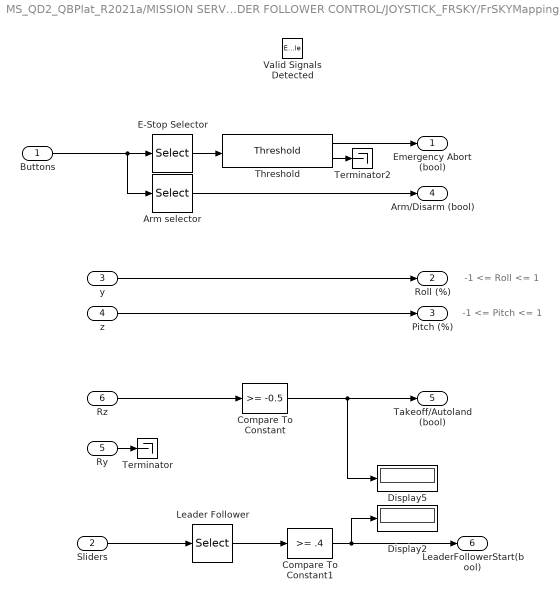
== system MS_QD2_QBPlat_R2021a/MISSION SERVER LEADER FOLLOWER CONTROL/JOYSTICK_FRSKY/FrSKYMapping ==
  note: -1 <= Roll <= 1
  note: -1 <= Pitch <= 1
  Buttons : Inport
  Sliders : Inport  Port=2
  y : Inport  Port=3
  z : Inport  Port=4
  Ry : Inport  Port=5
  Rz : Inport  Port=6
  Valid Signals Detected : EnablePort
  Arm selector : Selector  InputPortWidth=32  IndexOptions=Index vector (dialog)  Indices=[2]  OutputSizes=1
  Compare To Constant : simulink/Logic and Bit Operations/Compare To Constant  relop=>=  const=-0.5  OutDataTypeStr=boolean
  Compare To Constant1 : simulink/Logic and Bit Operations/Compare To Constant  relop=>=  const=.4  OutDataTypeStr=boolean
  Display2 : Display
  Display5 : Display
  E-Stop Selector : Selector  InputPortWidth=32  IndexOptions=Index vector (dialog)  Indices=[1]  OutputSizes=1
  Leader Follower : Selector  InputPortWidth=2  IndexOptions=Index vector (dialog)  Indices=[1]  OutputSizes=1
  Terminator : Terminator
  Terminator2 : Terminator
  Threshold : quarc_library/Discontinuities/Threshold  operator=>=  param_src=Specify via dialog  threshold=0.5  duration=0.2
      settings: SourceProductName=QUARC Targets
  Emergency Abort (bool) : Outport  VectorParamsAs1DForOutWhenUnconnected=off
  Roll (%) : Outport  Port=2  VectorParamsAs1DForOutWhenUnconnected=off
  Pitch (%) : Outport  Port=3  VectorParamsAs1DForOutWhenUnconnected=off
  "Arm/Disarm (bool) " : Outport  Port=4  VectorParamsAs1DForOutWhenUnconnected=off
  Takeoff/Autoland (bool) : Outport  Port=5  VectorParamsAs1DForOutWhenUnconnected=off
  LeaderFollowerStart(bool) : Outport  Port=6  VectorParamsAs1DForOutWhenUnconnected=off
  wires:
  Buttons/1 -> Arm selector/1, E-Stop Selector/1
  Arm selector/1 -> "Arm/Disarm (bool) "/1
  y/1 -> Roll (%)/1
  z/1 -> Pitch (%)/1
  Rz/1 -> Compare To Constant/1
  Sliders/1 -> Leader Follower/1
  E-Stop Selector/1 -> Threshold/1
  Compare To Constant/1 -> Takeoff/Autoland (bool)/1, Display5/1
  Threshold/1 -> Emergency Abort (bool)/1
  Threshold/2 -> Terminator2/1
  Leader Follower/1 -> Compare To Constant1/1
  Compare To Constant1/1 -> Display2/1, LeaderFollowerStart(bool)/1
  Ry/1 -> Terminator/1
